simulink model "iksolvermodel"  (R2024b)
settings: Solver=VariableStepAuto  StartTime=0.0  StopTime=10.0  RelTol=1e-3
settings Model: Creator=sinan  LastModifiedBy=sinan

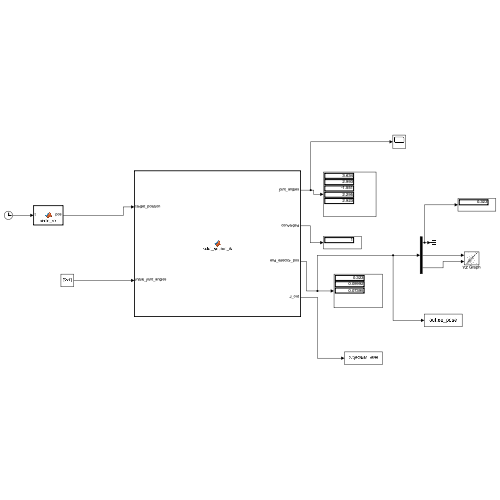
[thumbnail: Simulink's stored preview of the top-level diagram]
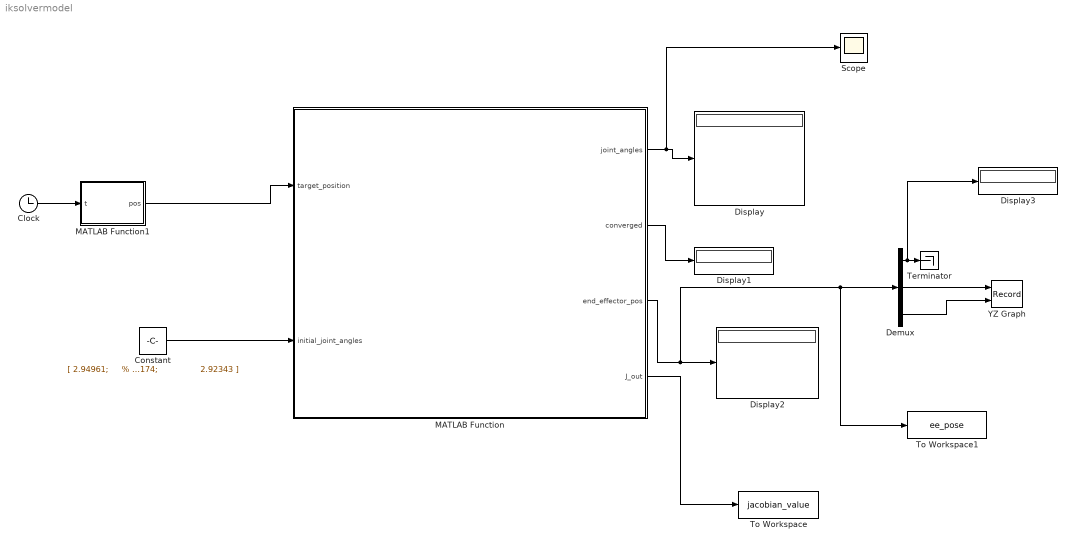
== system iksolvermodel ==
  Clock : Clock
  Constant : Constant  Value=|
      | [ 2.94961;     % eklem ofsetleri [rad]
      |                2.70526;
      |               -2.54818;
      |                3.36174;
      |                2.92343 ]
  Demux : Demux  Outputs=3
  Display{,1..3} (4 alike) : Display
  MATLAB Function : MATLAB Function  TreatAsAtomicUnit=on
  MATLAB Function1 : MATLAB Function  TreatAsAtomicUnit=on
  Scope : Scope
  Terminator : Terminator
  To Workspace : ToWorkspace  VariableName=jacobian_value  SaveFormat=Timeseries  SampleTime=-1
  To Workspace1 : ToWorkspace  VariableName=ee_pose  SaveFormat=Timeseries  SampleTime=-1
  YZ Graph : Record  FileSettingsInternal="{\"entries\":[{\"content\":{\"excelSettings\":{\"content\":{},\"type\":\"Streamout.ExcelSettings\"}},\"type\":\"Streamout.FileSettingStorage\",\"uuid\":\"\"}],\"packageUris\":[\"http:\\/\\/schema.mathworks.com\\/mf0\\/streamout_blocks\\/R2020a\"],\"version\":\"1.0\"}"  Layout=[1 1]  SignalsInternal="{\"entries\":[{\"content\":{\"signals\":[{\"content\":{\"blockPath\":[],\"dimensions\":[1,1],\"domain\":\"\",\"lineColor\":\"#a2142f\",\"plots\":[ 1 ],\"port\":1,\"sid\":[\"\"],\"signalID\":1,\"signalName\":\"Demux:2\"},\"type\":\"RecordBlkView.Signal\",\"uuid\":\"\"},{\"content\":{\"blockPath\":[],\"dimensions\":[1,1],\"domain\":\"\",\"lineColor\":\"#139fff\",\"plots\":[ 1 ],\"port\":2,\"sid\":[\"\"],\"signalID\":2,\"signalName\":\"Demux:3\"},\"type\":\"RecordBlkView.Signal\",\"uuid\":\"\"}]},\"type\":\"RecordBlkView.InputSignals\",\"uuid\":\"\"}],\"packageUris\":[\"http:\\/\\/schema.mathworks.com\\/mf0\\/streamout_blocks\\/R2020a\"],\"version\":\"1.0\"}"  VisualizationBindings="{\"xyplotplugin\":{\"info\":[{\"series\":[{\"bindingParametersList\":[{\"parameter\":\"X-Axis\",\"signalID\":1,\"signalName\":\"Demux:2\"},{\"parameter\":\"Y-Axis\",\"signalID\":2,\"signalName\":\"Demux:3\"}],\"seriesID\":0}],\"subplotID\":1}]}}"  CompatibilityTag=XY
  wires:
  Constant/1 -> MATLAB Function/2(initial_joint_angles)
  MATLAB Function/1(joint_angles) -> Scope/1, Display/1
  MATLAB Function/2(converged) -> Display1/1
  MATLAB Function/3(end_effector_pos) -> To Workspace1/1, Demux/1, Display2/1
  MATLAB Function/4(J_out) -> To Workspace/1
  Clock/1 -> MATLAB Function1/1(t)
  MATLAB Function1/1(pos) -> MATLAB Function/1(target_position)
  Demux/2 -> YZ Graph/1
  Demux/3 -> YZ Graph/2
  Demux/1 -> Display3/1, Terminator/1

== matlab function iksolvermodel/MATLAB Function1 ==
  data: t input; pos output
function pos = circle_ref(t)
%#codegen   % Simulink Uygunluğu
R     = 0.10;          % yarıçap [m]
Trev  = 5;             % 1 tur süresi [s]
w     = 2*pi/Trev;     % açısal hız [rad/s]
x0    = 0.323;         % sabit x [m]
z0    = 0.074;         % daire merkezi z [m]

y =  R * cos(w*t);
z =  z0 + R * sin(w*t);
pos = [x0; y; z];      % 3×1 hedef pozisyonu
end

== matlab function iksolvermodel/MATLAB Function ==
  data: target_position input; joint_angles output; initial_joint_angles input; converged output; end_effector_pos output; J_out output
function [joint_angles, converged, end_effector_pos, J_out] = kuka_youbot_ik( ...
                                   target_position, initial_joint_angles)
%#codegen   % Simulink / Embedded Coder uyum etiketi

%% Sabitler
MAX_ITER = int32(1000);
EPS_POS  = 1e-4;
ALPHA    = 0.10;
OFFSETS  = [ 2.94961;
             2.70526;
            -2.54818;
             3.36174;
             2.92343 ];

%% Başlangıç
joint_angles = initial_joint_angles;   % 5×1
converged    = false;
target_p     = target_position(:);     % 3×1

%% İteratif IK
for k = int32(1):MAX_ITER
    T_current = forward_kinematics(joint_angles, OFFSETS);
    cur_p     = T_current(1:3,4);
    err       = target_p - cur_p;

    if norm(err) < EPS_POS
        converged = true;
        break;
    end

    J      = compute_jacobian(joint_angles, OFFSETS);
    dtheta = ALPHA * pinv(J(1:3,:)) * err;   % yalnızca pozisyonel kısım
    joint_angles = joint_angles + dtheta;
end

%% Nihai çıktılar
T_ee              = forward_kinematics(joint_angles, OFFSETS); % 4×4
end_effector_pos  = T_ee(1:3,4);                              % 3×1
J_out             = compute_jacobian(joint_angles, OFFSETS);  % 6×5
end   % ===== Ana fonksiyon sonu =====


%% -------------------------------------------------
function T = forward_kinematics(q, OFF)
DH = [ 0.033,  pi/2,  0.147,  q(1)+OFF(1);
       0.155,  0,     0,      q(2)+OFF(2);
       0.135,  0,     0,      q(3)+OFF(3);
       0,      pi/2,  0,      q(4)+OFF(4);
       0,      0,     0.2174, q(5)+OFF(5) ];
T = eye(4);
for i = 1:5
    T = T * dh_matrix(DH(i,1), DH(i,2), DH(i,3), DH(i,4));
end
end


function J = compute_jacobian(q, OFF)
DH = [ 0.033,  pi/2,  0.147,  q(1)+OFF(1);
       0.155,  0,     0,      q(2)+OFF(2);
       0.135,  0,     0,      q(3)+OFF(3);
       0,      pi/2,  0,      q(4)+OFF(4);
       0,      0,     0.2174, q(5)+OFF(5) ];

T   = eye(4);
Ts  = zeros(4,4,6);                % sabit boyut
Ts(:,:,1) = T;

for i = 1:5
    T = T * dh_matrix(DH(i,1), DH(i,2), DH(i,3), DH(i,4));
    Ts(:,:,i+1) = T;
end

pe = T(1:3,4);
J  = zeros(6,5);

for i = 1:5
    z   = Ts(1:3,3,i);
    p   = Ts(1:3,4,i);
    J(1:3,i) = cross(z, pe - p);   % lineer kısım
    J(4:6,i) = z;                  % açısal kısım
end
end


function T = dh_matrix(a, alpha, d, theta)
T = [cos(theta), -sin(theta)*cos(alpha),  sin(theta)*sin(alpha), a*cos(theta);
     sin(theta),  cos(theta)*cos(alpha), -cos(theta)*sin(alpha), a*sin(theta);
     0,           sin(alpha),             cos(alpha),            d;
     0,           0,                     0,                     1];
end
